simulink model "Glideslope"  (Simulink 5.0)
settings: Solver=ode45  StartTime=0.0  StopTime=10.0  MaxStep=1e-3  RelTol=1e-12  AbsTol=1e-12
values from neighbouring files (symbols this model uses):
  alpha_trim = u(1)    [DOTRIM.M]
  T_trim = u(2)    [DOTRIM.M]
undefined symbols (not defined in the file or in its folder): magnitude
settings Model: LastModifiedBy=Administrator

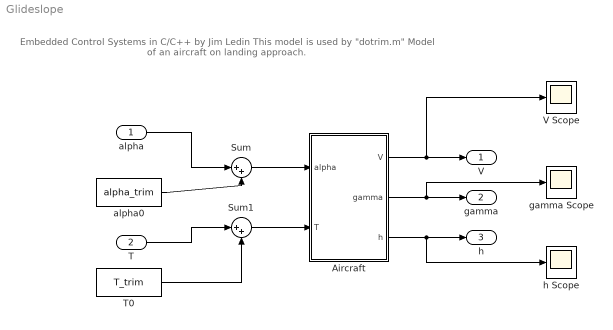
== system Glideslope ==
  note: Embedded Control Systems in C/C++
      | by Jim Ledin
      |
      | This model is used by "dotrim.m"
      |
      | Model of an aircraft on landing approach.
  alpha : Inport
  T : Inport  Port=2
  Aircraft : Subsystem
  Sum : Sum  Inputs=|++  SaturateOnIntegerOverflow=on
  Sum1 : Sum  Inputs=|++  SaturateOnIntegerOverflow=on
  T0 : Constant  Value=T_trim
  V Scope : Scope
      settings: TimeRange=10  YMin=81.8  YMax=81.8
  alpha0 : Constant  Value=alpha_trim
  gamma Scope : Scope
      settings: TimeRange=10  YMin=-0.0523599  YMax=-0.0523599
  h Scope : Scope
      settings: TimeRange=10  YMin=-8e-010  YMax=0  SaveName=ScopeData2
  V : Outport
  gamma : Outport  Port=2
  h : Outport  Port=3
  wires:
  Aircraft/1(V) -> V/1, V Scope/1
  Aircraft/2(gamma) -> gamma/1, gamma Scope/1
  Aircraft/3(h) -> h/1, h Scope/1
  alpha/1 -> Sum/1
  Sum/1 -> Aircraft/1(alpha)
  T/1 -> Sum1/1
  Sum1/1 -> Aircraft/2(T)
  alpha0/1 -> Sum/2
  T0/1 -> Sum1/2

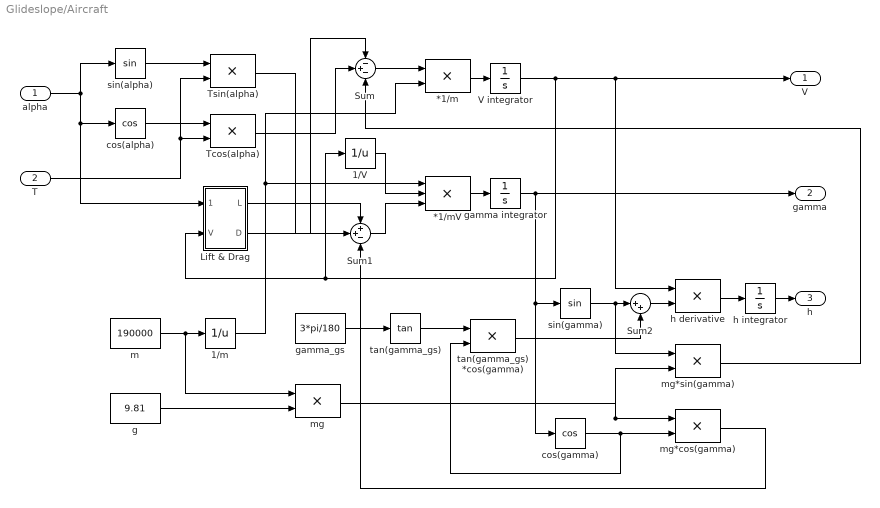
== system Glideslope/Aircraft ==
  alpha : Inport
  T : Inport  Port=2
  *1/m : Product  SaturateOnIntegerOverflow=on
  *1/mV : Product  Inputs=3  SaturateOnIntegerOverflow=on
  1/V : Math  Operator=reciprocal
  1/m : Math  Operator=reciprocal
  Lift & Drag : Subsystem
  Sum : Sum  Inputs=-+-  SaturateOnIntegerOverflow=on
  Sum1 : Sum  Inputs=++-  SaturateOnIntegerOverflow=on
  Sum2 : Sum  Inputs=|++  SaturateOnIntegerOverflow=on
  "Tcos(alpha) " : Product  SaturateOnIntegerOverflow=on
  "Tsin(alpha) " : Product  SaturateOnIntegerOverflow=on
  V integrator : Integrator  InitialCondition=81.8
  cos(alpha) : Trigonometry  Operator=cos
  cos(gamma) : Trigonometry  Operator=cos
  g : Constant  Value=9.81
  gamma integrator : Integrator  InitialCondition=-3*pi/180
  gamma_gs : Constant  Value=3*pi/180
  h integrator : Integrator
  "h derivative " : Product  SaturateOnIntegerOverflow=on
  m : Constant  Value=190000
  mg : Product  SaturateOnIntegerOverflow=on
  mg*cos(gamma) : Product  SaturateOnIntegerOverflow=on
  mg*sin(gamma) : Product  SaturateOnIntegerOverflow=on
  sin(alpha) : Trigonometry
  sin(gamma) : Trigonometry
  tan(gamma_gs) : Trigonometry  Operator=tan
  tan(gamma_gs) *cos(gamma) : Product  SaturateOnIntegerOverflow=on
  V : Outport
  gamma : Outport  Port=2
  h : Outport  Port=3
  wires:
  m/1 -> 1/m/1, mg/1
  V integrator/1 -> V/1, "h derivative "/1, Lift & Drag/2(V), 1/V/1
  gamma integrator/1 -> gamma/1, sin(gamma)/1, cos(gamma)/1
  h integrator/1 -> h/1
  "h derivative "/1 -> h integrator/1
  sin(gamma)/1 -> mg*sin(gamma)/1, Sum2/1
  alpha/1 -> Lift & Drag/1(alpha), cos(alpha)/1, sin(alpha)/1
  sin(alpha)/1 -> "Tsin(alpha) "/1
  cos(alpha)/1 -> "Tcos(alpha) "/1
  T/1 -> "Tcos(alpha) "/2, "Tsin(alpha) "/2
  g/1 -> mg/2
  mg/1 -> mg*sin(gamma)/2, mg*cos(gamma)/1
  cos(gamma)/1 -> mg*cos(gamma)/2, tan(gamma_gs) *cos(gamma)/2
  *1/m/1 -> V integrator/1
  1/m/1 -> *1/m/2, *1/mV/1
  Sum/1 -> *1/m/1
  Lift & Drag/2(D) -> Sum/1
  "Tcos(alpha) "/1 -> Sum/2
  mg*sin(gamma)/1 -> Sum/3
  Lift & Drag/1(L) -> Sum1/1
  "Tsin(alpha) "/1 -> Sum1/2
  mg*cos(gamma)/1 -> Sum1/3
  1/V/1 -> *1/mV/2
  *1/mV/1 -> gamma integrator/1
  Sum1/1 -> *1/mV/3
  gamma_gs/1 -> tan(gamma_gs)/1
  Sum2/1 -> "h derivative "/2
  tan(gamma_gs)/1 -> tan(gamma_gs) *cos(gamma)/1
  tan(gamma_gs) *cos(gamma)/1 -> Sum2/2

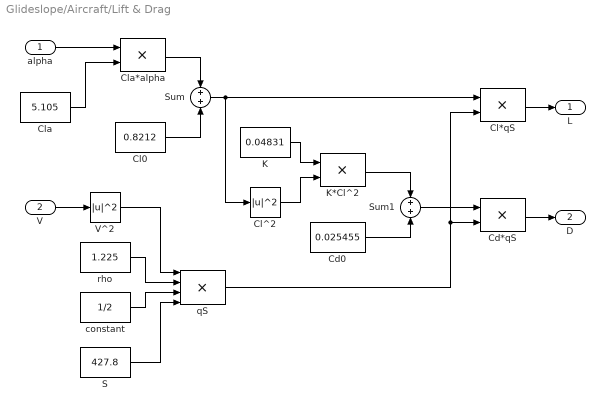
== system Glideslope/Aircraft/Lift & Drag ==
  alpha : Inport
  V : Inport  Port=2
  Cd*qS : Product  SaturateOnIntegerOverflow=on
  Cd0 : Constant  Value=0.025455
  Cl*qS : Product  SaturateOnIntegerOverflow=on
  Cl0 : Constant  Value=0.8212
  Cl^2 : Math  Operator=magnitude^2
  Cla : Constant  Value=5.105
  Cla*alpha : Product  SaturateOnIntegerOverflow=on
  K : Constant  Value=0.04831
  K*Cl^2 : Product  SaturateOnIntegerOverflow=on
  S : Constant  Value=427.8
  Sum : Sum  Inputs=+|+  SaturateOnIntegerOverflow=on
  Sum1 : Sum  Inputs=+|+  SaturateOnIntegerOverflow=on
  V^2 : Math  Operator=magnitude^2
  constant : Constant  Value=1/2
  qS : Product  Inputs=4  SaturateOnIntegerOverflow=on
  rho : Constant  Value=1.225
  L : Outport
  D : Outport  Port=2
  wires:
  Cla/1 -> Cla*alpha/2
  Cla*alpha/1 -> Sum/1
  Cl0/1 -> Sum/2
  Sum/1 -> Cl^2/1, Cl*qS/1
  K*Cl^2/1 -> Sum1/1
  Cd0/1 -> Sum1/2
  alpha/1 -> Cla*alpha/1
  V/1 -> V^2/1
  constant/1 -> qS/3
  V^2/1 -> qS/1
  S/1 -> qS/4
  rho/1 -> qS/2
  Cl*qS/1 -> L/1
  Sum1/1 -> Cd*qS/1
  Cd*qS/1 -> D/1
  qS/1 -> Cd*qS/2, Cl*qS/2
  Cl^2/1 -> K*Cl^2/2
  K/1 -> K*Cl^2/1
